simulink subsystem "Create_LLA_from_States"  (R2022b)
settings: Solver=VariableStepAuto  StartTime=0.0  StopTime=10.0  RelTol=1e-3
undefined symbols (not defined in the file): Earth, ref_height, ref_lat, ref_lon, WGS84
libraries: aerolibtransform2 x1
settings Model: Creator=The MathWorks, Inc.  LastModifiedBy=The MathWorks, Inc.
settings SolverCC: AlgebraicLoopSolver=TrustRegion  MaxZcPerStep=1
settings DebuggingCC: UnconnectedInputMsg=warning  UnconnectedOutputMsg=warning  UnconnectedLineMsg=warning  SFMachineParentedDataDiag=warning
settings ModelReferenceCC: EnableRefExpFcnMdlSchedulingChecks=on
settings RTWCC: DLArmComputeVersion=19.05

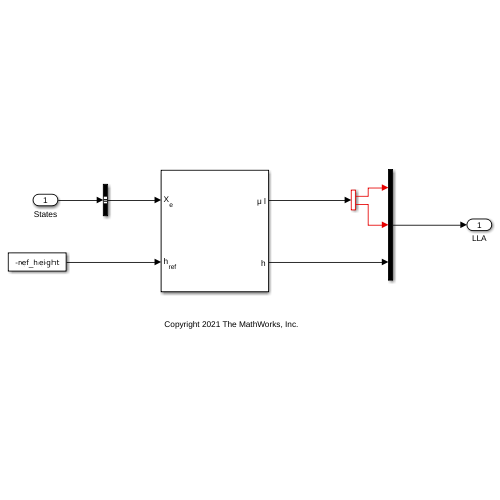
[thumbnail: Simulink's stored preview of the top-level diagram]
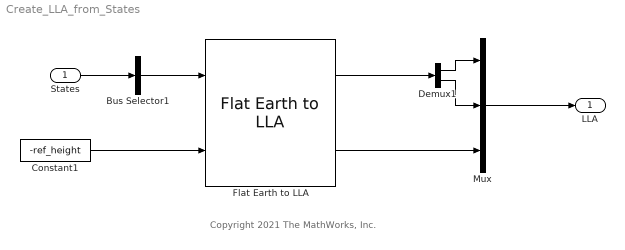
== system Create_LLA_from_States ==
  note: Copyright 2021 The MathWorks, Inc.
  States : Inport
  Bus Selector1 : BusSelector  OutputSignals=X,Y,Z  OutputAsBus=on
  Constant1 : Constant  Value=-ref_height  OutDataTypeStr=Inherit: Inherit via back propagation  SampleTime=-1
  Demux1 : Demux  Outputs=2
  Flat Earth to LLA : aerolibtransform2/Flat Earth to LLA  units=Metric (MKS)  ptype=Earth (WGS84)  F=1/298.257223563  R=6378137  refPosPort=off  LL0=[ref_lat ref_lon]  psi=0
  Mux : Mux  Inputs=3
  LLA : Outport
  wires:
  Flat Earth to LLA/1 -> Demux1/1
  Flat Earth to LLA/2 -> Mux/3
  Mux/1 -> LLA/1
  States/1 -> Bus Selector1/1
  Constant1/1 -> Flat Earth to LLA/2
  Demux1/2 -> Mux/2
  Demux1/1 -> Mux/1
  Bus Selector1/1 -> Flat Earth to LLA/1
